simulink model "Inverter_SS"  (R2020b)
settings: Solver=VariableStepAuto  StartTime=0.0  StopTime=10.0  RelTol=1e-3
libraries: PB_Library_Master x1
settings Model: Creator=gfretti  LastModifiedBy=nbutler2
settings SFSimCC: CustomCodeUndefinedFunction=UseInterfaceOnly

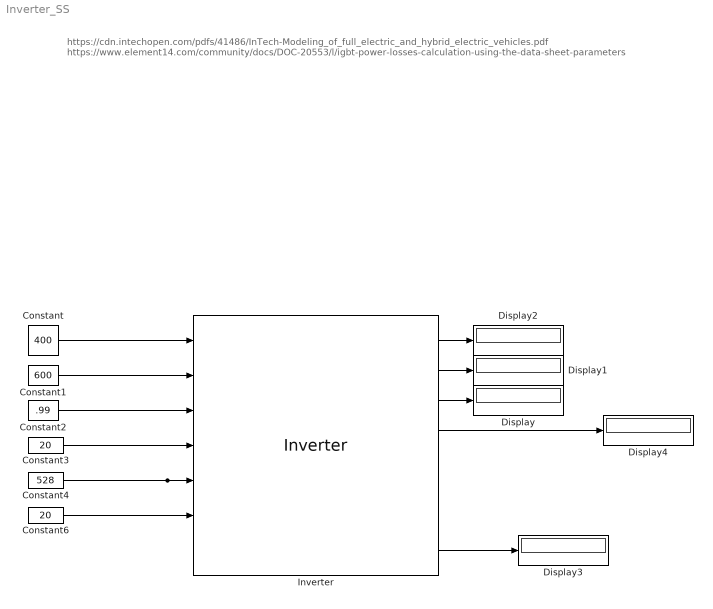
== system Inverter_SS ==
  note: https://cdn.intechopen.com/pdfs/41486/InTech-Modeling_of_full_electric_and_hybrid_electric_vehicles.pdf
      |
      | https://www.element14.com/community/docs/DOC-20553/l/igbt-power-losses-calculation-using-the-data-sheet-parameters
  Constant : Constant  Value=400
  Constant1 : Constant  Value=600
  Constant2 : Constant  Value=.99
  Constant3 : Constant  Value=20
  Constant4 : Constant  Value=528
  Constant6 : Constant  Value=20
  Display{,1..4} (5 alike) : Display
  Inverter : PB_Library_Master/Inverter  T_M=[25 175]  u_D_M=[0.9375 0.957142857142856]  u_ce0_M=[0.911764705882352 0.789473684210528]  R_c_M=[0.0588235294117647 0.105263157894737]  R_D_M=[0.0625 0.0571428571428572]  E0_M=[6.8e-05 6.8e-05]  E1_M=[5.68e-05 5.68e-05]  f_sw_M=20000  L_s_M=0.1  P_max_I=500  V_phase_I=600  f_sw_I=0  L_s_I=0.1
  wires:
  Constant/1 -> Inverter/1
  Constant1/1 -> Inverter/2
  Constant2/1 -> Inverter/3
  Constant3/1 -> Inverter/4
  Constant4/1 -> Inverter/5
  Constant6/1 -> Inverter/6
  Inverter/2 -> Display1/1
  Inverter/3 -> Display/1
  Inverter/1 -> Display2/1
  Inverter/8 -> Display3/1
  Inverter/4 -> Display4/1
